simulink model "dwc_primarydcdc"  (R2020b)
settings: Solver=VariableStepAuto  StartTime=0.0  StopTime=0.6  FixedStep=t_step
undefined symbols (not defined in the file): C1, C2, Cb, f_opt, Ion, k, ki_1, kp_1, L1, L2, Lb, Lithium, M, R, R1, R2, R_load, Rb, t_step, Vl, Vs
libraries: powerlib x36, powerlib_meascontrol x2, electricdrivelib x1, eePowerMeasurement x1
settings Model: Creator=Chuanyue Li  LastModifiedBy=kjaku
settings DataIOCC: ReturnWorkspaceOutputs=off
settings DebuggingCC: ArithmeticOperatorsInVariantConditions=warning
settings SFSimCC: SimUseLocalCustomCode=off  CustomCodeUndefinedFunction=UseInterfaceOnly
settings RTWCC: RTWUseLocalCustomCode=off

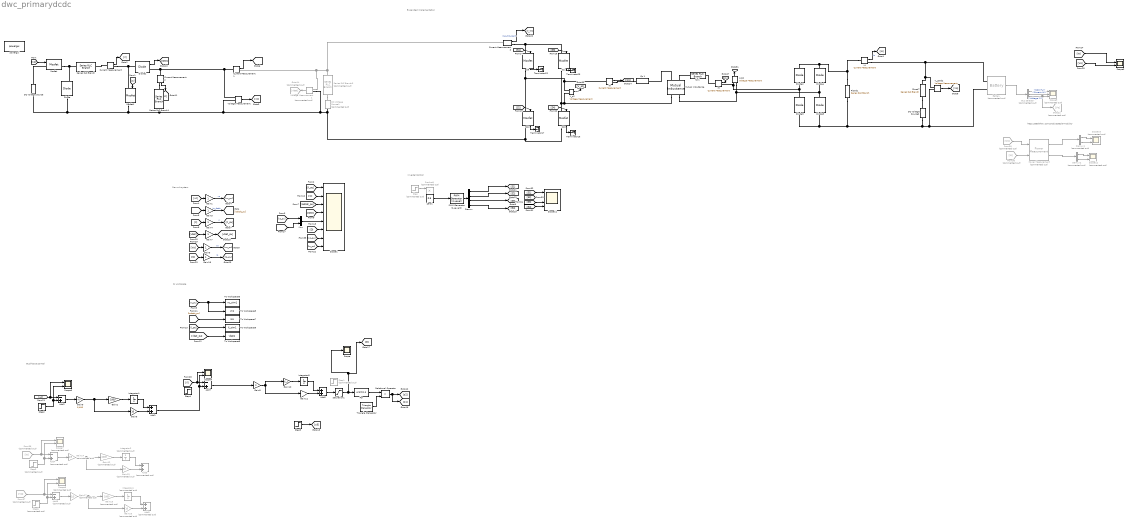
== system dwc_primarydcdc ==
  note: https://stealthev.com/product/tesla-module/
  note: to workspace
  note: Per unit system
  note: Buck-boost control
  note: Expanded implementation
  note: Inverter Control
  Add1 : Sum
  Add2 : Sum  Inputs=-+
  Add3 : Sum  Commented=on
  Add4 : Sum  Commented=on  Inputs=-+
  Add5 : Sum  Commented=on
  Add6 : Sum
  Add7 : Sum  Inputs=-+
  Add8 : Sum  Commented=on  Inputs=-+
  Battery : electricdrivelib/Extra Sources/Battery  Commented=on  BatType=Lithium-Ion  ShowTempParam=off  ThermalPreset=no  ShowAgeParam=off  NomV=22.8  NomQ=230  SOC=50  Batt_Tr=30  PresetModel=on  MaxQ=230  MinV=17.1  FullV=26.5389  Dis_rate=100  R=0.0009913  Normal_OP=208  expZone="[24.6328         11.3]"  current=[6.5 13 32.5]  Units=Time  Tci=20  NomT=20  T2=-30  MaxQ2=4.8  FullV2=7.1  Normal_OP2=5.655  expZone2="[6.58           1]"  Rca=0.6  ti=2000  Dp=0  Neq0=0  Tsim=1e6  Ta1=25  Qeol=5.4*0.9  Reol=0.013333*1.2  Char_age=[2.3478, 3]  Dis_age=[2.3478, 10]  N1=1500  N2=10500  N3=1000  N4=1400  Ta2=45  N5=950
  Bus Selector : BusSelector  Commented=on  OutputSignals=SOC (%),Current (A),Voltage (V)
  Cp 1 : powerlib/Elements/Series RLC Branch  LConnTagsString=__new0  RConnTagsString=__new0  BranchType=C  Resistance=R  Inductance=1e-3  SetiL0=off  InitialCurrent=0  Capacitance=C1  Setx0=off  InitialVoltage=0  Measurements=None
  Cs 1 : powerlib/Elements/Series RLC Branch  LConnTagsString=__new0  RConnTagsString=__new0  BranchType=C  Resistance=R  Inductance=1e-3  SetiL0=off  InitialCurrent=0  Capacitance=C2  Setx0=off  InitialVoltage=0  Measurements=None
  Current Measurement{,1..3} (4 alike) : powerlib/Measurements/Current Measurement  PhasorSimulation=off  OutputType=Complex  PSBequivalent=0
  DC Voltage Source : powerlib/Electrical Sources/DC Voltage Source  Amplitude=Vs  Measurements=None
  DC Voltage Source1 : powerlib/Electrical Sources/DC Voltage Source  Commented=on  Amplitude=Vl  Measurements=None
  DC Voltage Source2 : powerlib/Electrical Sources/DC Voltage Source  Amplitude=400  Measurements=None
  Demux : Demux
  Demux1 : Demux  Commented=on  Outputs=2
  Demux2 : Demux  Commented=on  Outputs=2
  Diode : powerlib/Power Electronics/Diode  Ron=0.001  Lon=0  Vf=0  IC=0  UseSnubber=0  Rs=500000  Cs=250e-9  Measurements=on
  Diode1 : powerlib/Power Electronics/Diode  Ron=0.001  Lon=0  Vf=0  IC=0  UseSnubber=0  Rs=500000  Cs=250e-9  Measurements=on
  Diode{2..5} (4 alike) : powerlib/Power Electronics/Diode  Ron=0.001  Lon=0  Vf=0.8  IC=0  UseSnubber=0  Rs=500  Cs=250e-9  Measurements=off
  Fcn : Fcn  Expr=u(1)*2-1
  From30 : From  Commented=on  GotoTag=Io
  From36 : From  Commented=on  GotoTag=Io
  From37 : From  Commented=on  GotoTag=Vo
  From38 : From  Commented=on  GotoTag=Vo
  Gain{1,3..5,7,18} (6 alike) : Gain
  Gain10 : Gain  Gain=ki_1
  Gain11 : Gain  Gain=kp_1
  Gain12 : Gain  Commented=on  Gain=1000
  Gain13 : Gain  Commented=on  Gain=10
  Gain14 : Gain  Commented=on  Gain=1/5
  Gain15 : Gain  Commented=on  Gain=1000
  Gain16 : Gain  Commented=on  Gain=10
  Gain17 : Gain  Commented=on  Gain=1/5
  Gain2 : Gain  Gain=1000
  Gain6 : Gain  Gain=10
  Gain8 : Gain  Gain=k
  Gain9 : Gain  Gain=1/400
  Goto14 : Goto  Commented=on  GotoTag=vbat
  Goto22 : Goto  Commented=on  GotoTag=Vo
  I4 : powerlib/Measurements/Current Measurement  PhasorSimulation=off  OutputType=Complex  PSBequivalent=0
  I8 : powerlib/Measurements/Current Measurement  PhasorSimulation=off  OutputType=Complex  PSBequivalent=0
  I9 : powerlib/Measurements/Current Measurement  PhasorSimulation=off  OutputType=Complex  PSBequivalent=0
  Integrator1 : Integrator
  Integrator2 : Integrator  Commented=on
  Integrator3 : Integrator
  Integrator4 : Integrator  Commented=on
  Mosfet : powerlib/Power Electronics/Mosfet  Ron=0.01  Lon=0  Rd=0.01  Vfd=0  IC=0  Rs=1e5  Cs=inf  Measurements=on
  Mosfet1 : powerlib/Power Electronics/Mosfet  Ron=0.01  Lon=0  Rd=0.01  Vfd=0  IC=0  Rs=1e5  Cs=inf  Measurements=on
  Mutual Inductance : powerlib/Elements/Mutual Inductance  LConnTagsString=a|b  RConnTagsString=A|B  TypeOfMutual=Two or three windings with equal mutual terms  NumberOfWindings=3  SelfImpedance1=[R1 L1]  SelfImpedance2=[R2 L2]  ThreeWindings=off  SelfImpedance3=[ 1.1 1.1e-03]  MutualImpedance=[0 M*2]  InductanceMatrix="[1.0 0.9  0.9 ;  0.9 1.0  0.9;  0.9 0.9 1.0 ] * 1e-3"  ResistanceMatrix="[1.0 0.9  0.9 ;  0.9 1.0  0.9;  0.9 0.9 1.0 ]"  Measurements=None
      settings: AttributesFormatString=\n  SourceProductBaseCode=PS
  Mux : Mux  Inputs=2
  PWM Generator (2-Level)2 : powerlib_meascontrol/Pulse & Signal Generators/PWM Generator (2-Level)  ModulatorType=Single-phase full-bridge - Bipolar modulation (4 pulses)  ModulatorMode=Unsynchronized  Fc=f_opt  Pc=90  nF=27  MinMax="[ 0  1 ]"  SamplingTechnique=Natural  ModulatingSignals=off  m=0.8  Freq=60  Phase=0  Ts=0  ShowCarrierOutport=off
  Power Measurement : eePowerMeasurement/Power Measurement  Commented=on  LabelModeActiveChoice=Continuous  F=f_opt*2  K=[0 1]  Ts=0
      settings: SourceProductBaseCode=PS
  Product1 : Product  Commented=on
  Relational Operator : RelationalOperator  Operator=>  OutDataTypeStr=boolean  RndMeth=Zero
  Rload1 : powerlib/Elements/Series RLC Branch  LConnTagsString=__new0  RConnTagsString=__new0  BranchType=C  Resistance=R_load  Inductance=1e-3  SetiL0=off  InitialCurrent=0  Capacitance=100e-6  Setx0=on  InitialVoltage=Vb  Measurements=None
  Rload7 : powerlib/Elements/Series RLC Branch  LConnTagsString=__new0  RConnTagsString=__new0  BranchType=R  Resistance=R_load*0+Rb  Inductance=1e-3  SetiL0=off  InitialCurrent=0  Capacitance=10e-6  Setx0=on  InitialVoltage=300  Measurements=None
  S{9..12} (4 alike) : powerlib/Power Electronics/Mosfet  Ron=0.1  Lon=0  Rd=Rds  Vfd=0  IC=0  Rs=1e5  Cs=inf  Measurements=on
  Saturation1 : Saturate  UpperLimit=0.95  LowerLimit=-1
  Scope : Scope
  Scope1 : Scope  NumInputPorts=8
  Scope{7..8,10,12} (4 alike) : Scope  Commented=on  NumInputPorts=2
  Scope11 : Scope  NumInputPorts=4
  Scope3 : Scope  NumInputPorts=2
  Scope4 : Scope  NumInputPorts=2
  Scope6 : Scope  NumInputPorts=2
  Scope9 : Scope  Commented=on  NumInputPorts=3
  Series RLC Branch : powerlib/Elements/Series RLC Branch  LConnTagsString=__new0  RConnTagsString=__new0  BranchType=L  Resistance=1  Inductance=Lb  SetiL0=off  InitialCurrent=10  Capacitance=1e-6  Setx0=off  InitialVoltage=0  Measurements=None
  Series RLC Branch1 : powerlib/Elements/Series RLC Branch  LConnTagsString=__new0  RConnTagsString=__new0  BranchType=C  Resistance=1  Inductance=1e-3  SetiL0=off  InitialCurrent=0  Capacitance=Cb  Setx0=off  InitialVoltage=400  Measurements=None
  Series RLC Branch3 : powerlib/Elements/Series RLC Branch  Commented=on  LConnTagsString=__new0  RConnTagsString=__new0  BranchType=R  Resistance=Rb  Inductance=Lb  SetiL0=off  InitialCurrent=0  Capacitance=1e-6  Setx0=off  InitialVoltage=0  Measurements=None
  Step : Step  Commented=on  Time=0.05  Before=0.3  After=0.35  SampleTime=0
  Step1 : Step  Commented=on  Time=0.3  Before=0.45  After=0.5  SampleTime=0
  Step2 : Step  Time=0.2  Before=410  After=415  SampleTime=0
  Step3 : Step  Commented=on  Time=0.3  Before=5  After=5.5  SampleTime=0
  Step4 : Step  Time=0.3  Before=25  After=30  SampleTime=0
  Step5 : Step  Time=0.05  Before=1  SampleTime=0
  Step6 : Step  Commented=on  Before=410  After=410  SampleTime=0
  Terminator{16..17,22..23} (4 alike) : Terminator
  To Workspace5 : ToWorkspace  VariableName=vc1  SaveFormat=Timeseries  SampleTime=-1
  To Workspace6 : ToWorkspace  VariableName=vc_sim1  SaveFormat=Timeseries  SampleTime=-1
  To Workspace7 : ToWorkspace  VariableName=io1  SaveFormat=Timeseries  SampleTime=-1
  To Workspace8 : ToWorkspace  VariableName=vbat1  SaveFormat=Timeseries  SampleTime=-1
  To Workspace9 : ToWorkspace  VariableName=Il_sim1  SaveFormat=Timeseries  SampleTime=-1
  Triangle Generator : powerlib_meascontrol/Pulse & Signal Generators/Triangle Generator  Freq=s_fre  Phase=0  Ts=0
  V_Load2 : powerlib/Measurements/Voltage Measurement  PhasorSimulation=off  OutputType=Complex  PSBequivalent=0
  V_S2 : powerlib/Measurements/Voltage Measurement  PhasorSimulation=off  OutputType=Complex  PSBequivalent=0
  V_p2 : powerlib/Measurements/Voltage Measurement  PhasorSimulation=off  OutputType=Complex  PSBequivalent=0
  Voltage Measurement : powerlib/Measurements/Voltage Measurement  PhasorSimulation=off  OutputType=Complex  PSBequivalent=0
  Voltage Measurement1 : powerlib/Measurements/Voltage Measurement  Commented=on  PhasorSimulation=off  OutputType=Complex  PSBequivalent=0
  Zero1 : Constant  Value=0.5  OutDataTypeStr=Inherit: Inherit via back propagation
  powergui : powerlib/powergui  Priority=1  SimulationMode=Continuous  SampleTime=t_step  frequency=60  Iterations=50  frequencyindice=0  Pbase=100e6  ErrMax=1e-4  UnitsV=kV  UnitsW=MW  buscounter=0  FunctionMessages=off  echomessages=off  EnableUseOfTLC=off  CurrentSourceSwitches=off  DisableSnubberDevices=off  DisableRonSwitches=off  DisableVfSwitches=off  DisplayEquations=off  AutomaticDiscreteSolvers=off  SolverType=Tustin/Backward Euler (TBE)  Interpol=off  ExternalGateDelay=off  methode=off  Ts=100  x0status=blocks  SPID=off  SwTol=0  HookPort=off  NonlinearTolerance=1e-4  nMaxIteration=100  ContinueOnMaxIteration=off  RestoreLinks=warning  ResistiveCurrentMeasurement=off  Frange=[0:2:500]  Ylog=off  Xlog=on  ShowGrid=off  save=off  variable=ZData  structure=logsout  ZoomFFT=off  StartTime=0.2  cycles=10  DisplayStyle=2  fundamental=50  FreqAxis=off  MaxFrequency=1000  frequencyindicesteady=1  RmsSteady=1  display=off
  wires:
  [s1] -> Mosfet/1
  [s2] -> Mosfet1/1
  Current Measurement/1 -> [il]
  Voltage Measurement/1 -> [vc]
  [il_pu] -> Scope1/1
  [vc] -> Gain1/1
  Gain1/1 -> [vc_pu]  "vc"
  [io_dcdc] -> Gain3/1
  Current Measurement1/1 -> [io_dcdc]
  Gain3/1 -> [iodcdc_pu]  "io_dcdc"
  [iodcdc_pu] -> Scope1/3
  Gain4/1 -> [il_pu]  "il"
  [il] -> Gain4/1
  Diode1/1 -> [iDIO]
  [iDIO] -> Scope1/4
  Current Measurement2/1 -> [ic]
  [ic] -> Scope1/2
  Voltage Measurement1/1 -> Goto14/1
  [vbat] -> Gain7/1
  Gain7/1 -> [vbat_pu]
  [vc_pu] -> Mux/1
  Mux/1 -> Scope1/5
  [vbat_pu] -> Mux/2
  Triangle Generator/1 -> Relational Operator/2
  Fcn/1 -> Relational Operator/1
  Relational Operator/1 -> [s1], [s2]
  Step5/1 -> [s3]
  Add6/1 -> Saturation1/1
  Integrator3/1 -> Add6/1
  Gain11/1 -> Add6/2
  Saturation1/1 -> [D], Scope/1, Fcn/1
  [il] -> Scope4/1, Add7/1
  Gain10/1 -> Integrator3/1
  Gain8/1 -> Gain11/1, Gain10/1
  Add1/1 -> Scope4/2, Add7/2
  [D] -> Scope1/6
  Add7/1 -> Gain8/1
  [vc_pu] -> To Workspace5/1, To Workspace6/1
  [iodcdc_pu] -> To Workspace7/1
  [vbat_pu] -> To Workspace8/1
  [il_pu] -> To Workspace9/1
  Demux/4 -> [S4]
  I4/1 -> [Io]  "Io"
  [S3] -> Scope11/3
  Demux/3 -> [S3]
  [S4] -> S10/1
  I8/1 -> [Ip1]
  Demux/1 -> [S1]
  [S2] -> Scope11/2
  S12/1 -> Terminator17/1
  S11/1 -> Terminator23/1
  [S4] -> Scope11/4
  S10/1 -> Terminator16/1
  Current Measurement3/1 -> [I_in]  "Input Current"
  [S2] -> S12/1
  S9/1 -> Terminator22/1
  [S3] -> S11/1
  V_Load2/1 -> [Vo]
  V_p2/1 -> [V_p1]
  [S1] -> Scope11/1
  PWM Generator (2-Level)2/1 -> Demux/1
  Demux/2 -> [S2]
  V_S2/1 -> [Vs1]
  Step/1 -> Product1/1
  [S1] -> S9/1
  I9/1 -> [Is1]
  Zero1/1 -> PWM Generator (2-Level)2/1
  [Io] -> Scope3/1
  [Vo] -> Scope3/2
  [Vo] -> Gain5/1
  Gain5/1 -> [vo_pu]  "vo"
  [vo_pu] -> Scope1/7
  Gain9/1 -> Gain6/1, Gain2/1
  Gain2/1 -> Integrator1/1
  Gain6/1 -> Add1/2
  Integrator1/1 -> Add1/1
  [vc] -> Scope6/1, Add2/1
  Add2/1 -> Gain9/1
  Step2/1 -> Scope6/2, Add2/2
  Step3/1 -> Add4/2, Scope7/2
  Add4/1 -> Gain14/1
  From36/1 -> Add4/1, Scope7/1
  Integrator2/1 -> Add3/1
  Gain13/1 -> Add3/2
  Gain12/1 -> Integrator2/1
  Gain14/1 -> Gain12/1, Gain13/1
  Gain17/1 -> Gain16/1, Gain15/1
  Gain15/1 -> Integrator4/1
  Gain16/1 -> Add5/2
  Integrator4/1 -> Add5/1
  From37/1 -> Scope8/1, Add8/1
  Add8/1 -> Gain17/1
  Step6/1 -> Scope8/2, Add8/2
  Battery/1 -> Bus Selector/1
  Bus Selector/1 -> Scope9/1  "<SOC (%)>"
  Bus Selector/2 -> Scope9/2  "<Current (A)>"
  Bus Selector/3 -> Goto22/1, Scope9/3  "<Voltage (V)>"
  From30/1 -> Power Measurement/2
  From38/1 -> Power Measurement/1
  Power Measurement/1 -> Demux1/1
  Power Measurement/2 -> Demux2/1
  Demux1/1 -> Scope10/1
  Demux1/2 -> Scope10/2
  Demux2/2 -> Scope12/2
  Demux2/1 -> Scope12/1
  [io_pu] -> Scope1/8
  [Io] -> Gain18/1
  Gain18/1 -> [io_pu]  "io"
  connections:
  DC Voltage Source/RConn1 -- Mosfet/LConn1
  Mosfet/RConn1 -- Diode/RConn1 -- Series RLC Branch/LConn1
  Mosfet1/LConn1 -- Current Measurement/RConn1 -- Diode1/LConn1
  S10/RConn1 -- Series RLC Branch1/RConn1 -- DC Voltage Source/LConn1 -- Diode/LConn1 -- Mosfet1/RConn1 -- Voltage Measurement/LConn2 -- Voltage Measurement1/LConn2 -- DC Voltage Source1/LConn1 -- S12/RConn1
  Current Measurement/LConn1 -- Series RLC Branch/RConn1
  Current Measurement2/RConn1 -- Series RLC Branch1/LConn1
  Series RLC Branch3/LConn1 -- DC Voltage Source1/RConn1
  Diode5/LConn1 -- Diode3/LConn1 -- V_Load2/LConn2 -- Battery/LConn2 -- DC Voltage Source2/LConn1 -- Rload1/RConn1
  Mutual Inductance/RConn1 -- V_p2/LConn2 -- S11/RConn1 -- S10/LConn1
  Diode2/LConn1 -- Diode3/RConn1 -- V_S2/LConn1 -- I9/RConn1
  Current Measurement3/RConn1 -- S11/LConn1 -- S9/LConn1
  V_p2/LConn1 -- S9/RConn1 -- S12/LConn1 -- I8/LConn1
  V_S2/LConn2 -- Diode4/LConn1 -- Diode5/RConn1 -- Mutual Inductance/RConn2
  V_Load2/LConn1 -- Battery/LConn1 -- I4/RConn1 -- Rload7/LConn1
  I8/RConn1 -- Cp 1/RConn1
  Cs 1/LConn1 -- Mutual Inductance/LConn2
  I9/LConn1 -- Cs 1/RConn1
  Mutual Inductance/LConn1 -- Cp 1/LConn1
  Rload7/RConn1 -- DC Voltage Source2/RConn1
  Current Measurement1/LConn1 -- Current Measurement2/LConn1 -- Diode1/RConn1 -- Voltage Measurement/LConn1
  Voltage Measurement1/LConn1 -- Current Measurement1/RConn1 -- Current Measurement3/LConn1 -- Series RLC Branch3/RConn1
  I4/LConn1 -- Rload1/LConn1 -- Diode2/RConn1 -- Diode4/RConn1
